simulink model "h175_model_cathode_harness_hctrl_basic"  (R2023a)
settings: Solver=VariableStepAuto  StartTime=0.0  StopTime=4750  RelTol=1e-2
InitFcn:
  | run("cathode_subsystem_parameters.m")
undefined symbols (not defined in the file or in its folder): sigbuilder_block
libraries: nesl_utility x12, fl_lib x10, simulink x5, slpidlib x2, eeGeneralControl x2, VariableTimeLowPassFilter x1
(part 1 of 2)
settings Model: Creator=adrian.taveras  LastModifiedBy=stefan.notter
settings SolverCC: MaxConsecutiveMinStep=20  ZeroCrossAlgorithm=Adaptive  DecoupledContinuousIntegration=on
settings DataIOCC: Refine=2
settings OptimizationCC: ReuseModelBlockBuffer=off
settings DebuggingCC: IgnoredZcDiagnostic=none
settings SimscapeCC: SimscapeLogType=all

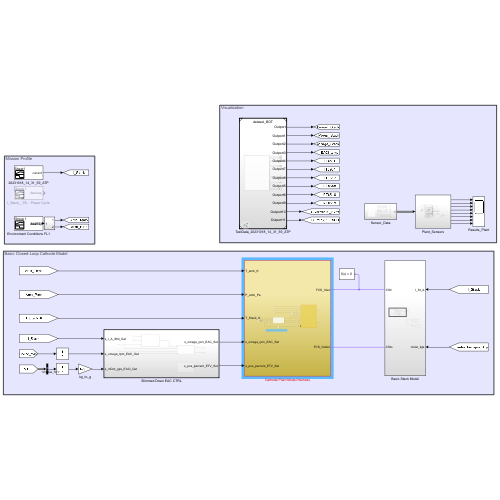
[thumbnail: Simulink's stored preview of the top-level diagram]
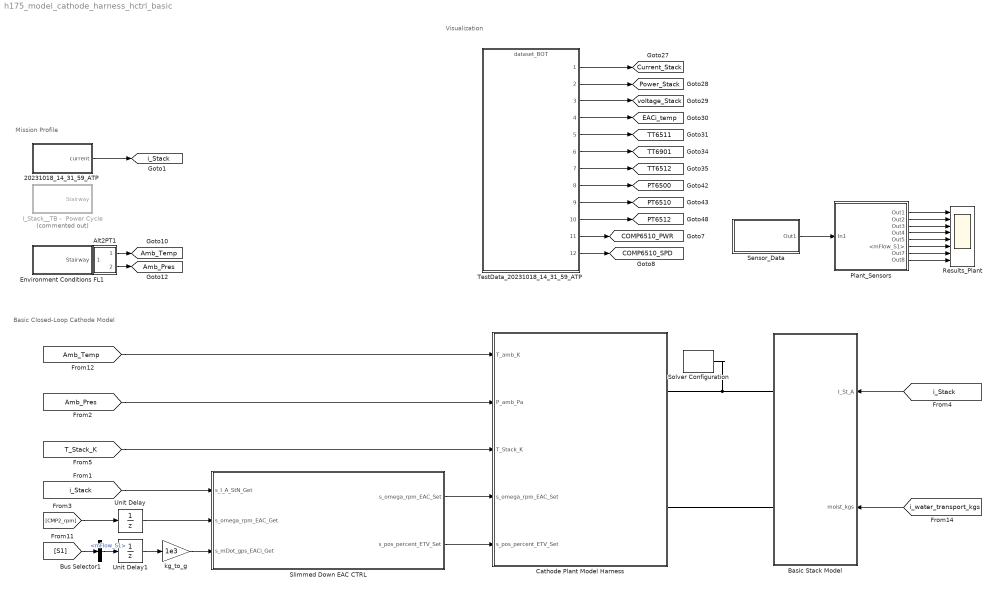
== system h175_model_cathode_harness_hctrl_basic ==
  note: Basic Closed-Loop Cathode Model
  note: Visualization
  note: Mission Profile
  20231018_14_31_59_ATP : Subsystem  Tag=STV Subsys  LoadFcn=sigbuilder_block('load');  StartFcn=sigbuilder_block('start');  StopFcn=sigbuilder_block('stop');  ClipboardFcn=sigbuilder_block('clipboard');  mask(Sigbuilder block){tuvar=[0:10]}
      mask help: Simulink:masks:SigbuilderBlock_MD
      mask init:
      | if ~strcmp(get_param(bdroot(gcbh),'SimulationStatus'),'stopped') tuvar = sigbuilder_block('maskInit'); end
      settings: CopyFcn=sigbuilder_block('copy');  DeleteFcn=sigbuilder_block('delete');  ModelCloseFcn=sigbuilder_block('modelClose');  PreSaveFcn=sigbuilder_block('preSave');  PauseFcn=sigbuilder_block('pause');  ContinueFcn=sigbuilder_block('continue');  NameChangeFcn=sigbuilder_block('namechange');  OpenFcn=sigbuilder_block('open',[725.25 330.75 938.25 556.5 ]);  CloseFcn=sigbuilder_block('close');
      mask Display: plot(0, 0, 100, 100,[2, 2, 32, 32, 2], [68, 8, 8, 68, 68],[32, 2], [38, 38], [32, 19, 2],[53, 60, 44], [32, 17, 17, 2],[16, 16, 31, 31]);txt = getActiveGroup(gcbh);text(2, 100, txt,'verticalAlignment', 'top');
  Alt2PT1 : Subsystem
  Basic Stack Model : Subsystem
      settings: PortSchema="{\"entries\":[{\"content\":{\"sides\":[{\"content\":{\"connectorIds\":[\"LConn1\",\"LConn2\"]},\"type\":\"ConnectorPlacement.EquallySpacedRectSide\",\"uuid\":\"19460938-b288-4d21-b4cd-9dae603c1776\"},{\"content\":{\"connectorIds\":[\"In1\",\"In2\"],\"side\":\"RIGHT\"},\"type\":\"ConnectorPlacement.EquallySpacedRectSide\",\"uuid\":\"f9fd6515-5c99-4012-9e0e-a9d1faf30c36\"},{\"content\":{\"side\":\"TOP\"},\"type\":\"ConnectorPlacement.EquallySpacedRectSide\",\"uuid\":\"36dd5767-135b-4114-983d-9ffe53efa4e0\"}]},\"type\":\"ConnectorPlacement.EquallySpacedConnector\",\"uuid\":\"78d4a12b-2c5e-427b-baa6-4f95f1f393d1\"}],\"packageUris\":[\"http://schema.mathworks.com/mf0/Connector/R2020b\"],\"version\":\"1.0\"}"
  Bus Selector1 : BusSelector  OutputSignals=mFlow_S1
  Cathode Plant Model Harness : Subsystem
  Environment Conditions FL1 : Subsystem  Tag=STV Subsys  LoadFcn=sigbuilder_block('load',[5.4 5.4 1141.2 580.8 ]);  StartFcn=sigbuilder_block('start');  StopFcn=sigbuilder_block('stop');  ClipboardFcn=sigbuilder_block('clipboard');  mask(Sigbuilder block){tuvar=[0:10]}
      mask help: Simulink:masks:SigbuilderBlock_MD
      mask init:
      | if ~strcmp(get_param(bdroot(gcbh),'SimulationStatus'),'stopped') tuvar = sigbuilder_block('maskInit'); end
      settings: CopyFcn=sigbuilder_block('copy');  DeleteFcn=sigbuilder_block('delete');  ModelCloseFcn=sigbuilder_block('modelClose');  PreSaveFcn=sigbuilder_block('preSave');  PauseFcn=sigbuilder_block('pause');  ContinueFcn=sigbuilder_block('continue');  NameChangeFcn=sigbuilder_block('namechange');  OpenFcn=sigbuilder_block('open',[6 30 1908 951.75 ]);  CloseFcn=sigbuilder_block('close');
      mask Display: plot(0, 0, 100, 100,[2, 2, 32, 32, 2], [68, 8, 8, 68, 68],[32, 2], [38, 38], [32, 19, 2],[53, 60, 44], [32, 17, 17, 2],[16, 16, 31, 31]);txt = getActiveGroup(gcbh);text(2, 100, txt,'verticalAlignment', 'top');
  I_Stack__TB -  Power Cycle : Subsystem  Tag=STV Subsys  Commented=on  LoadFcn=sigbuilder_block('load');  StartFcn=sigbuilder_block('start');  StopFcn=sigbuilder_block('stop');  ClipboardFcn=sigbuilder_block('clipboard');  mask(Sigbuilder block){tuvar=[0:10]}
      mask help: Simulink:masks:SigbuilderBlock_MD
      mask init:
      | if ~strcmp(get_param(bdroot(gcbh),'SimulationStatus'),'stopped') tuvar = sigbuilder_block('maskInit'); end
      settings: CopyFcn=sigbuilder_block('copy');  DeleteFcn=sigbuilder_block('delete');  ModelCloseFcn=sigbuilder_block('modelClose');  PreSaveFcn=sigbuilder_block('preSave');  PauseFcn=sigbuilder_block('pause');  ContinueFcn=sigbuilder_block('continue');  NameChangeFcn=sigbuilder_block('namechange');  OpenFcn=sigbuilder_block('open',[329.4 141 551.4 321 ]);  CloseFcn=sigbuilder_block('close');
      mask Display: plot(0, 0, 100, 100,[2, 2, 32, 32, 2], [68, 8, 8, 68, 68],[32, 2], [38, 38], [32, 19, 2],[53, 60, 44], [32, 17, 17, 2],[16, 16, 31, 31]);txt = getActiveGroup(gcbh);text(2, 100, txt,'verticalAlignment', 'top');
  Plant_Sensors : Subsystem
  Results_Plant : Scope  NumInputPorts=8
  Sensor_Data : Subsystem
  Slimmed Down EAC CTRL : Subsystem  TreatAsAtomicUnit=on
      settings: RTWFcnNameOpts=Use subsystem name  RTWFileNameOpts=Use subsystem name
  Solver Configuration : nesl_utility/Solver Configuration  PhysicalDomain=network_engine_domain  SubClassName=solver  LeftPortType=input  RightPortType=generic  Tones=[]  Harmonics=[]  SimulateNoise=off  Profile=off  UseLocalSampling=off  EnableSwitchedLinearOptims=on  FrequencyDomain=off  UseCCode=off  RelTol=0.001  AbsTol=0.001  MinStep=1e-09  ToWorkspace=off  RevertToSquareIcSolve=off  NumHomotopyIterations=100  PhasorMode=off  PhasorModeNumHarmonics=1  ConsistencySolver=NEWTON_XTOL_AFTER_FTOL  IndexReductionMethod=DerivativeReplacement  DoDC=off  ResidualTolerance=1e-09  ConsistencyTolSource=GLOBAL  ConsistencyAbsTol=0.01  ConsistencyRelTol=0.01  ConsistencyTolFactor=0.1  UseLocalSolver=off  LocalSolverChoice=NE_BACKWARD_EULER_ADVANCER  ResolveIndetEquations=on  FunctionEvalNumThread=1  LocalSolverSampleTime=0.001  DoFixedCost=off  MaxNonlinIter=3  MaxModeIter=2  ComputeImpulses=off  ImpulseIterations=2  LinearAlgebra=auto  LinearAlgebraNumThread=0  EquationFormulation=NE_TIME_EF  DelaysMemoryBudget=8096  AutomaticFiltering=on  FilteringTimeConstant=0.005  PartitionStorageMethod=AS_NEEDED  PartitionMemoryBudget=1024  PartitionMethod=ROBUST
  TestData_20231018_14_31_59_ATP : ModelReference  ModelNameDialog=dataset_BOT.slx  SimulationMode=Normal  ModelReferenceVersion=1.7
  Unit Delay : UnitDelay  SampleTime=-1  HasFrameUpgradeWarning=on
  Unit Delay1 : UnitDelay  SampleTime=-1  HasFrameUpgradeWarning=on
  kg_to_g : Gain  Gain=1e3
  tag scope: Amb_Pres=global, Amb_Temp=global, COMP6510_PWR=global, COMP6510_SPD=global, Current_Stack=global, EACi_temp=global, PT6500=global, PT6510=global, PT6512=global, Power_Stack=global, TT6511=global, TT6512=global, TT6901=global, i_Stack=global, voltage_Stack=global
  wires:
  Plant_Sensors/1(Out1) -> Results_Plant/1
  Plant_Sensors/2(Out2) -> Results_Plant/2
  Plant_Sensors/3(Out3) -> Results_Plant/3
  Plant_Sensors/4(Out4) -> Results_Plant/4
  Plant_Sensors/5(Out5) -> Results_Plant/5
  Plant_Sensors/6(<mFlow_S1>) -> Results_Plant/6
  Plant_Sensors/7(Out7) -> Results_Plant/7
  Plant_Sensors/8(Out8) -> Results_Plant/8
  Alt2PT1/2(Out2) -> [Amb_Pres]
  Environment Conditions FL1/1(Stairway) -> Alt2PT1/1(In1)
  Alt2PT1/1(Out1) -> [Amb_Temp]
  20231018_14_31_59_ATP/1(current) -> [i_Stack]
  Sensor_Data/1(Out1) -> Plant_Sensors/1(In1)
  TestData_20231018_14_31_59_ATP/1 -> [Current_Stack]
  TestData_20231018_14_31_59_ATP/2 -> [Power_Stack]
  TestData_20231018_14_31_59_ATP/3 -> [voltage_Stack]
  TestData_20231018_14_31_59_ATP/4 -> [EACi_temp]
  TestData_20231018_14_31_59_ATP/5 -> [TT6511]
  TestData_20231018_14_31_59_ATP/6 -> [TT6901]
  TestData_20231018_14_31_59_ATP/7 -> [TT6512]
  TestData_20231018_14_31_59_ATP/11 -> [COMP6510_PWR]
  TestData_20231018_14_31_59_ATP/12 -> [COMP6510_SPD]
  TestData_20231018_14_31_59_ATP/10 -> [PT6512]
  TestData_20231018_14_31_59_ATP/9 -> [PT6510]
  TestData_20231018_14_31_59_ATP/8 -> [PT6500]
  [i_Stack] -> Basic Stack Model/1(I_St_A)
  [i_water_transport_kgs] -> Basic Stack Model/2(moist_kgs)
  [Amb_Temp] -> Cathode Plant Model Harness/1(T_amb_K)
  [Amb_Pres] -> Cathode Plant Model Harness/2(P_amb_Pa)
  Slimmed Down EAC CTRL/1(s_omega_rpm_EAC_Set) -> Cathode Plant Model Harness/4(s_omega_rpm_EAC_Set)
  Slimmed Down EAC CTRL/2(s_pos_percent_ETV_Set) -> Cathode Plant Model Harness/5(s_pos_percent_ETV_Set)
  [i_Stack] -> Slimmed Down EAC CTRL/1(s_I_A_StN_Get)
  [CMP2_rpm] -> Unit Delay/1
  [S1] -> Bus Selector1/1
  Bus Selector1/1 -> Unit Delay1/1  "<mFlow_S1>"
  kg_to_g/1 -> Slimmed Down EAC CTRL/3(s_mDot_gps_EACi_Get)
  Unit Delay/1 -> Slimmed Down EAC CTRL/2(s_omega_rpm_EAC_Get)
  Unit Delay1/1 -> kg_to_g/1
  [T_Stack_K] -> Cathode Plant Model Harness/3(T_Stack_K)
  connections:
  Solver Configuration/RConn1 -- Basic Stack Model/LConn1 -- Cathode Plant Model Harness/RConn1
  Basic Stack Model/LConn2 -- Cathode Plant Model Harness/RConn2

== system h175_model_cathode_harness_hctrl_basic/20231018_14_31_59_ATP ==
  Demux : Demux  Tag=STV Demux  Outputs=1
      settings: DisplayOption=none
  FromWs : FromWorkspace  Tag=STV FromWs  VariableName=tuvar
      SigBuilderData=|
      | common.afterFinalStr = 'Extrapolate'
      | common.sampleTime = 0
      | dataSet.timeRange = [0 4735]
      | dataSet.name = 'Sheet1'
      | sbobj.Groups.Name = 'Sheet1'
      | sbobj.Groups.Signals.Name = 'current'
      | sbobj.Groups.Signals.XData = [0 710 730 830 850 1000 1020 1080 1100 1200 1230 1260 1270 1320 1340 1390 1405 1455 1475 1525 1565 3990 4000 4030 4090 4130 4245 4270 4345 4355 4385 4395 4735]
      | sbobj.Groups.Signals.YData = [5 5 45 45 100 100 200 200 300 300 45 45 50 50 200 200 300 300 100 100 420 420 340 420 260 340 340 50 50 45 45 5 5]
      | sbobj.Groups.TimeRange = [0 4735]
  current : Outport  Tag=STV Outport
  wires:
  Demux/1 -> current/1
  FromWs/1 -> Demux/1

== system h175_model_cathode_harness_hctrl_basic/Alt2PT1 ==
  In1 : Inport
  Add1 : Sum  Inputs=-+
  Constant4 : Constant  Value=0.0065
  Constant5 : Constant  Value=288.15
  Constant6 : Constant  Value=101330
  Constant7 : Constant  Value=4.256
  Constant8 : Constant  Value=288.15
  Divide1 : Product  Inputs=*/
  Math Function1 : Math  Operator=pow
  Product2 : Product
  Product3 : Product
  Out1 : Outport
  Out2 : Outport  Port=2
  wires:
  Constant5/1 -> Divide1/2
  Constant8/1 -> Add1/2
  In1/1 -> Product2/1
  Add1/1 -> Out1/1, Divide1/1
  Constant4/1 -> Product2/2
  Math Function1/1 -> Product3/1
  Constant7/1 -> Math Function1/2
  Divide1/1 -> Math Function1/1
  Product2/1 -> Add1/1
  Constant6/1 -> Product3/2
  Product3/1 -> Out2/1

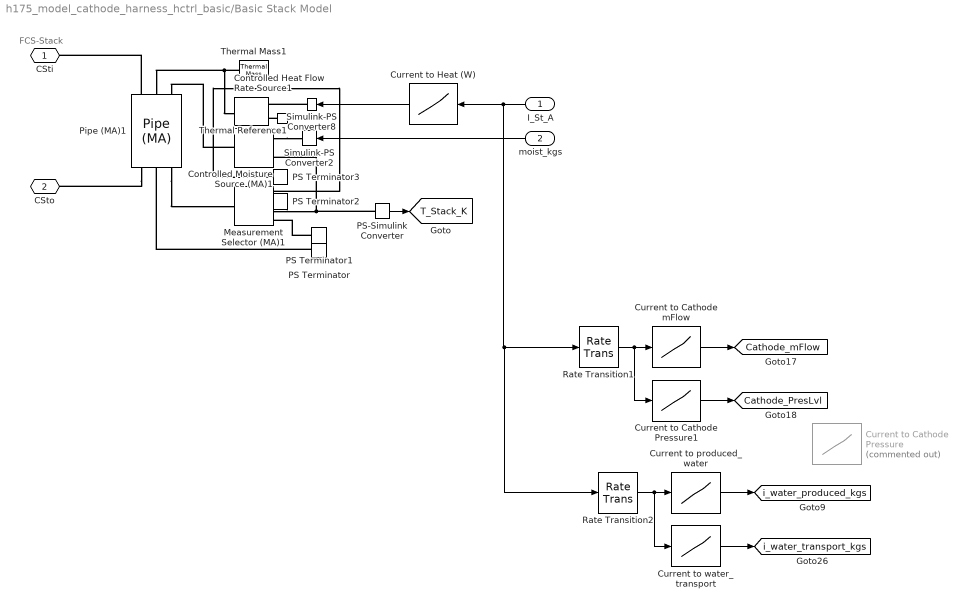
== system h175_model_cathode_harness_hctrl_basic/Basic Stack Model ==
  note: FCS-Stack
  I_St_A : Inport
  moist_kgs : Inport  Port=2
  Controlled Heat Flow Rate Source1 : fl_lib/Thermal/Thermal Sources/Controlled Heat Flow Rate Source
  Controlled Moisture Source (MA)1 : fl_lib/Moist Air/Sources/Moisture & Trace Gas Sources/Controlled Moisture Source (MA)  moisture_source_spec=foundation.enum.moisture_source_spec.vapor  Phi_S_specify=off  Phi_S_priority=None  Phi_S=0 kW  Phi_S_nominal_specify=off  Phi_S_nominal_unit=kW  Phi_S_nominal_value=1  mdot_w_S_specify=off  mdot_w_S_priority=None  mdot_w_S=0 kg/s  mdot_w_S_nominal_specify=off  mdot_w_S_nominal_unit=kg/s  mdot_w_S_nominal_value=1
      settings: InternalSimscapePortConfiguration="{\"Bottom\":[],\"Left\":[{\"id\":\"S\",\"label\":\"S\",\"type\":\"foundation.moist_air.moist_air_source\"}],\"Right\":[{\"id\":\"M\",\"label\":\"M\",\"type\":\"input\"},{\"id\":\"T\",\"label\":\"T\",\"type\":\"input\"}],\"Top\":[]}"
  Current to Cathode Pressure : Lookup_n-D  Commented=on  NumberOfTableDimensions=1  BreakpointsForDimension1=[0;50;100;150;200;250;300;350;400;510;600]  Table=[101330;110000;115000;125000;130000;140000;150000;165000;180000;200000;230000]  InternalRulePriority=Speed  RndMeth=Simplest
  Current to Cathode Pressure1 : Lookup_n-D  NumberOfTableDimensions=1  BreakpointsForDimension1=[0;50;100;150;200;250;300;350;400;510;600]  Table=[101330;140000;150000;175000;185000;195000;202500;210000;220000;235000;250000]  InternalRulePriority=Speed  RndMeth=Simplest
  Current to Cathode mFlow : Lookup_n-D  NumberOfTableDimensions=1  BreakpointsForDimension1=[0;50;100;150;200;250;300;350;400;510;600]  Table=[0;0.01;0.0225;0.035;0.045;0.055;0.068;0.0825;0.1;0.135;0.167]  InternalRulePriority=Speed  RndMeth=Simplest
  Current to Heat (W) : Lookup_n-D  NumberOfTableDimensions=1  BreakpointsForDimension1=[0:50:400]  Table=[0, 9932, 21438, 33442,47123, 59491, 77033, 93585, 112042]  InternalRulePriority=Speed  RndMeth=Simplest
  Current to produced_water : Lookup_n-D  NumberOfTableDimensions=1  BreakpointsForDimension1=[0;100;200;400;600]  Table=[0;6.491e-6;1.132e-5;1.762e-5;2.762e-5]  InternalRulePriority=Speed  RndMeth=Simplest
  Current to water_transport : Lookup_n-D  NumberOfTableDimensions=1  BreakpointsForDimension1=[0;100;200;400;600]  Table=[0;4.247e-3;8.494e-3;1.697e-2;2.548e-2]  InternalRulePriority=Speed  RndMeth=Simplest
  Measurement Selector (MA)1 : fl_lib/Moist Air/Sensors/Measurement Selector (MA)  moisture_spec=foundation.enum.moisture_spec.relative_humidity  trace_gas_spec=foundation.enum.trace_gas_spec.mole_fraction
  PS Terminator{,1..3} (4 alike) : fl_lib/Physical Signals/Sinks/PS Terminator
  PS-Simulink Converter : nesl_utility/PS-Simulink Converter  PhysicalDomain=network_engine_domain  SubClassName=ps_output  LeftPortType=input  RightPortType=output  PseudoPeriodic=off  Frequencies=[]  VectorFormat=inherit  Unit=inherit  AffineConversion=off
  Pipe (MA)1 : fl_lib/Moist Air/Elements/Pipe (MA)  length=1 m  area=1 m^2  Dh=.1 m  length_add=.1 m  roughness=15e-6 m  Re_lam=2000  Re_tur=4000  shape_factor=1  Nu_lam=3.66  wall_condensation=simscape.enum.onoff.on  RH_ws=1  time_constant=1e-3 s  moisture_trace_gas_source=foundation.enum.moisture_trace_gas_source.controlled  moisture_source_spec=foundation.enum.moisture_source_spec.vapor  moisture_mass_flow=0 kg/s  moisture_temperature_spec=foundation.enum.temperature_spec.atmospheric  moisture_temperature=293.15 K  trace_gas_mass_flow=0 kg/s  trace_gas_temperature_spec=foundation.enum.temperature_spec.atmospheric  trace_gas_temperature=293.15 K  p_I_specify=off  p_I_priority=High  p_I=0.101325 MPa  p_I_nominal_specify=off  p_I_nominal_unit=MPa  p_I_nominal_value=1  T_I_specify=off  T_I_priority=High  T_I=293.15 K  T_I_nominal_specify=off  T_I_nominal_unit=K  T_I_nominal_value=1  RH_I_specify=off  RH_I_priority=High  RH_I=0  RH_I_nominal_specify=off  RH_I_nominal_unit=1  RH_I_nominal_value=1  x_w_I_specify=off  x_w_I_priority=None  x_w_I=0  x_w_I_nominal_specify=off  x_w_I_nominal_unit=1  x_w_I_nominal_value=1  y_w_I_specify=off  y_w_I_priority=None  y_w_I=0  y_w_I_nominal_specify=off  y_w_I_nominal_unit=1  y_w_I_nominal_value=1  HR_I_specify=off  HR_I_priority=None  HR_I=0  HR_I_nominal_specify=off  HR_I_nominal_unit=1  HR_I_nominal_value=1  x_g_I_specify=off  x_g_I_priority=High  x_g_I=0  x_g_I_nominal_specify=off  x_g_I_nominal_unit=1  x_g_I_nominal_value=1  y_g_I_specify=off  y_g_I_priority=None  y_g_I=0  y_g_I_nominal_specify=off  y_g_I_nominal_unit=1  y_g_I_nominal_value=1
      settings: InternalSimscapePortConfiguration="{\"Bottom\":[],\"Left\":[{\"id\":\"A\",\"label\":\"A\",\"type\":\"foundation.moist_air.moist_air\"},{\"id\":\"H\",\"label\":\"H\",\"type\":\"foundation.thermal.thermal\"},{\"id\":\"S\",\"label\":\"S\",\"type\":\"foundation.moist_air.moist_air_source\"}],\"Right\":[{\"id\":\"B\",\"label\":\"B\",\"type\":\"foundation.moist_air.moist_air\"},{\"id\":\"W\",\"label\":\"W\",\"type\":\"output\"},{\"id\":\"F\",\"label\":\"F\",\"type\":\"output\"}],\"Top\":[]}"
  Rate Transition1 : RateTransition
  Rate Transition2 : RateTransition
  Simulink-PS Converter2 : nesl_utility/Simulink-PS Converter  PhysicalDomain=network_engine_domain  SubClassName=ps_input  LeftPortType=input  RightPortType=output  PseudoPeriodic=off  Frequencies=[]  NoiseDistribution=none  NoiseParameters=[]  Unit=1  AffineConversion=off  FilteringAndDerivatives=provide  SimscapeFilterOrder=1  InputFilterTimeConstant=0.001  UdotUserProvided=0
  Simulink-PS Converter8 : nesl_utility/Simulink-PS Converter  PhysicalDomain=network_engine_domain  SubClassName=ps_input  LeftPortType=input  RightPortType=output  PseudoPeriodic=off  Frequencies=[]  NoiseDistribution=none  NoiseParameters=[]  Unit=W  AffineConversion=off  FilteringAndDerivatives=provide  SimscapeFilterOrder=1  InputFilterTimeConstant=0.001  UdotUserProvided=0
  Thermal Mass1 : fl_lib/Thermal/Thermal Elements/Thermal Mass  mass_type=foundation.enum.constant_variable.constant  mass=10 kg  sp_heat=447 J/(K*kg)  mass_min=1e-6 kg  num_ports=foundation.enum.numPorts2.one  m_specify=off  m_priority=High  m=1 kg  m_nominal_specify=off  m_nominal_unit=kg  m_nominal_value=1  T_specify=off  T_priority=High  T=300 K  T_nominal_specify=off  T_nominal_unit=K  T_nominal_value=1  Q_specify=off  Q_priority=None  Q=0 W  Q_nominal_specify=off  Q_nominal_unit=W  Q_nominal_value=1
  Thermal Reference1 : fl_lib/Thermal/Thermal Elements/Thermal Reference
  CSti : PMIOPort  Side=Left
  CSto : PMIOPort  Port=2  Side=Left
  tag scope: Cathode_PresLvl=global, Cathode_mFlow=global, T_Stack_K=global, i_water_produced_kgs=global, i_water_transport_kgs=global
  wires:
  Current to Heat (W)/1 -> Simulink-PS Converter8/1
  moist_kgs/1 -> Simulink-PS Converter2/1
  I_St_A/1 -> Current to Heat (W)/1, Rate Transition2/1, Rate Transition1/1
  Rate Transition2/1 -> Current to water_transport/1, Current to produced_water/1
  Current to Cathode Pressure1/1 -> [Cathode_PresLvl]
  Current to water_transport/1 -> [i_water_transport_kgs]
  Rate Transition1/1 -> Current to Cathode Pressure1/1, Current to Cathode mFlow/1
  Current to Cathode mFlow/1 -> [Cathode_mFlow]
  Current to produced_water/1 -> [i_water_produced_kgs]
  PS-Simulink Converter/1 -> [T_Stack_K]
  connections:
  Measurement Selector (MA)1/RConn2 -- PS-Simulink Converter/LConn1 -- Controlled Moisture Source (MA)1/RConn2
  Thermal Mass1/LConn1 -- Controlled Heat Flow Rate Source1/LConn1 -- Pipe (MA)1/LConn2
  PS Terminator3/LConn1 -- Measurement Selector (MA)1/RConn4
  Thermal Reference1/LConn1 -- Controlled Heat Flow Rate Source1/RConn2
  Controlled Moisture Source (MA)1/RConn1 -- Simulink-PS Converter2/RConn1
  Pipe (MA)1/RConn3 -- Measurement Selector (MA)1/LConn1
  Controlled Moisture Source (MA)1/LConn1 -- Pipe (MA)1/LConn3
  Simulink-PS Converter8/RConn1 -- Controlled Heat Flow Rate Source1/RConn1
  Pipe (MA)1/LConn1 -- CSti/RConn1
  PS Terminator1/LConn1 -- Measurement Selector (MA)1/RConn1
  PS Terminator2/LConn1 -- Measurement Selector (MA)1/RConn3
  Pipe (MA)1/RConn1 -- CSto/RConn1
  PS Terminator/LConn1 -- Pipe (MA)1/RConn2

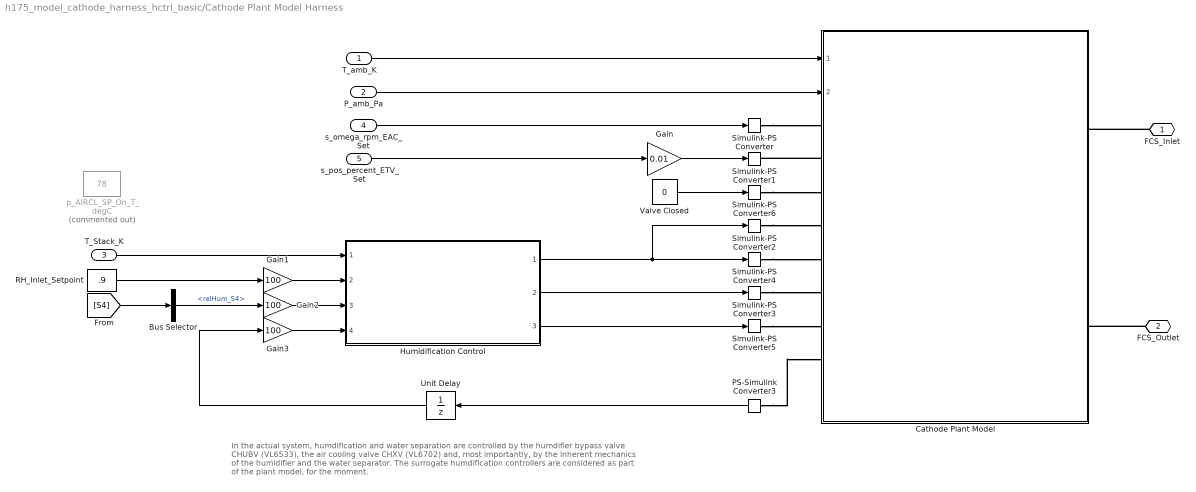
== system h175_model_cathode_harness_hctrl_basic/Cathode Plant Model Harness ==
  note: In the actual system, humdification and water separation are controlled by the humdifier bypass valve CHUBV (VL6533), the air cooling valve CHXV (VL6702) and, most importantly, by the inherent mechanics of the humidifier and the water separator.
      | The surrogate humdification controllers are considered as part of the plant model, for the moment.
  T_amb_K : Inport
  P_amb_Pa : Inport  Port=2
  T_Stack_K : Inport  Port=3
  s_omega_rpm_EAC_Set : Inport  Port=4
  s_pos_percent_ETV_Set : Inport  Port=5
  Bus Selector : BusSelector  OutputSignals=relHum_S4
  Cathode Plant Model : Subsystem  ReferencedSubsystem=cathode_subsystem_model
      settings: PortSchema="{\"entries\":[{\"content\":{\"sides\":[{\"content\":{\"connectorIds\":[\"In1\",\"In2\",\"LConn8\",\"LConn9\",\"LConn7\",\"LConn1\",\"LConn4\",\"LConn2\",\"LConn3\",\"LConn5\",\"LConn6\"]},\"type\":\"ConnectorPlacement.EquallySpacedRectSide\",\"uuid\":\"e3b30cb5-20d3-4977-927f-9fea068a9234\"},{\"content\":{\"connectorIds\":[\"RConn1\",\"RConn2\"],\"side\":\"RIGHT\"},\"type\":\"ConnectorPlacement.EquallySpacedRectSide\",\"uuid\":\"2d547627-9665-492a-afa4-fcc16b1173a1\"},{\"content\":{\"side\":\"TOP\"},\"type\":\"ConnectorPlacement.EquallySpacedRectSide\",\"uuid\":\"4ee6a80a-af1f-40b1-aa59-916ec7fe1294\"}]},\"type\":\"ConnectorPlacement.EquallySpacedConnector\",\"uuid\":\"0d82e4d1-cc18-4647-90fc-0df577891cdc\"}],\"packageUris\":[\"http://schema.mathworks.com/mf0/Connector/R2020b\"],\"version\":\"1.0\"}"
  Gain : Gain  Gain=0.01
  Gain1 : Gain  Gain=100
  Gain2 : Gain  Gain=100
  Gain3 : Gain  Gain=100
  Humidification Control : Subsystem  ReferencedSubsystem=cathode_subsystem_humdification
  PS-Simulink Converter3 : nesl_utility/PS-Simulink Converter  PhysicalDomain=network_engine_domain  SubClassName=ps_output  LeftPortType=input  RightPortType=output  PseudoPeriodic=off  Frequencies=[]  VectorFormat=inherit  Unit=inherit  AffineConversion=off
  RH_Inlet_Setpoint : Constant  Value=.9
  Simulink-PS Converter{,1..6} (7 alike) : nesl_utility/Simulink-PS Converter  PhysicalDomain=network_engine_domain  SubClassName=ps_input  LeftPortType=input  RightPortType=output  PseudoPeriodic=off  Frequencies=[]  NoiseDistribution=none  NoiseParameters=[]  Unit=1  AffineConversion=off  FilteringAndDerivatives=provide  SimscapeFilterOrder=1  InputFilterTimeConstant=0.001  UdotUserProvided=0
  Unit Delay : UnitDelay  SampleTime=-1  HasFrameUpgradeWarning=on
  Valve Closed : Constant  Value=0
  p_AIRCL_SP_On_T_degC : Constant  Commented=on  Value=78
  FCS_Inlet : PMIOPort  Side=Right
  FCS_Outlet : PMIOPort  Port=2  Side=Right
  wires:
  T_amb_K/1 -> Cathode Plant Model/1
  P_amb_Pa/1 -> Cathode Plant Model/2
  s_omega_rpm_EAC_Set/1 -> Simulink-PS Converter/1
  s_pos_percent_ETV_Set/1 -> Gain/1
  RH_Inlet_Setpoint/1 -> Gain1/1
  T_Stack_K/1 -> Humidification Control/1
  Gain/1 -> Simulink-PS Converter1/1
  Humidification Control/3 -> Simulink-PS Converter5/1
  Humidification Control/1 -> Simulink-PS Converter4/1, Simulink-PS Converter2/1
  Humidification Control/2 -> Simulink-PS Converter3/1
  Valve Closed/1 -> Simulink-PS Converter6/1
  Gain1/1 -> Humidification Control/2
  [S4] -> Bus Selector/1
  Bus Selector/1 -> Gain2/1  "<relHum_S4>"
  Gain2/1 -> Humidification Control/3
  PS-Simulink Converter3/1 -> Unit Delay/1
  Unit Delay/1 -> Gain3/1
  Gain3/1 -> Humidification Control/4
  connections:
  FCS_Inlet/RConn1 -- Cathode Plant Model/RConn1
  FCS_Outlet/RConn1 -- Cathode Plant Model/RConn2
  Simulink-PS Converter/RConn1 -- Cathode Plant Model/LConn8
  Cathode Plant Model/LConn9 -- Simulink-PS Converter1/RConn1
  Simulink-PS Converter6/RConn1 -- Cathode Plant Model/LConn7
  Simulink-PS Converter2/RConn1 -- Cathode Plant Model/LConn1
  Simulink-PS Converter3/RConn1 -- Cathode Plant Model/LConn2
  Simulink-PS Converter4/RConn1 -- Cathode Plant Model/LConn4
  Simulink-PS Converter5/RConn1 -- Cathode Plant Model/LConn3
  PS-Simulink Converter3/LConn1 -- Cathode Plant Model/LConn5

== system h175_model_cathode_harness_hctrl_basic/Environment Conditions FL1 ==
  Demux : Demux  Tag=STV Demux  Outputs=1
      settings: DisplayOption=none
  FromWs : FromWorkspace  Tag=STV FromWs  VariableName=tuvar
      SigBuilderData=|
      | common.afterFinalStr = 'Extrapolate'
      | common.sampleTime = 0
      | dataSet.timeRange = [0 22226]
      | dataSet.name = 'Group 1'
      | sbobj.Groups.Name = 'Group 1'
      | sbobj.Groups.Signals.Name = 'Stairway'
      | sbobj.Groups.Signals.XData = [0 1 1.1 1.2 1.3 120 270 670 1450 7450 7510 21146 21826 22226]
      | sbobj.Groups.Signals.YData = [0 0 0 0 0 0 250 650 1100 1100 1000 1000 500 0]
      | sbobj.Groups.TimeRange = [0 22226]
  Stairway : Outport  Tag=STV Outport
  wires:
  Demux/1 -> Stairway/1
  FromWs/1 -> Demux/1

== system h175_model_cathode_harness_hctrl_basic/I_Stack__TB -  Power Cycle ==
  Demux : Demux  Tag=STV Demux  Outputs=1
      settings: DisplayOption=none
  FromWs : FromWorkspace  Tag=STV FromWs  VariableName=tuvar
      SigBuilderData=|
      | common.afterFinalStr = 'Extrapolate'
      | common.sampleTime = 0
      | dataSet.timeRange = [0 600]
      | dataSet.name = 'Group 1'
      | sbobj.Groups.Name = 'Group 1'
      | sbobj.Groups.Signals.Name = 'Stairway'
      | sbobj.Groups.Signals.XData = [0 180 190 250 260 320 330 390 410 460 470 530 540 600]
      | sbobj.Groups.Signals.YData = [100 100 200 200 400 400 600 600 300 300 200 200 100 100]
      | sbobj.Groups.TimeRange = [0 600]
  Stairway : Outport  Tag=STV Outport
  wires:
  Demux/1 -> Stairway/1
  FromWs/1 -> Demux/1

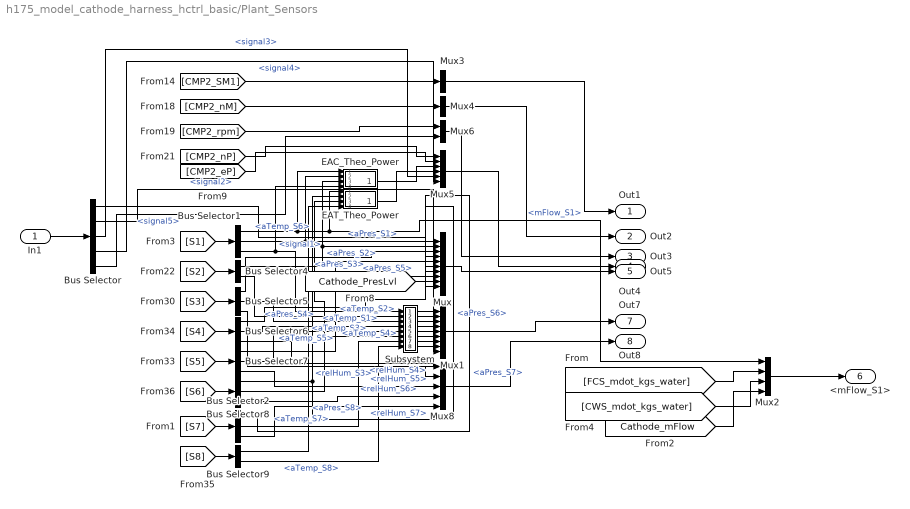
== system h175_model_cathode_harness_hctrl_basic/Plant_Sensors ==
  In1 : Inport
  Bus Selector : BusSelector  OutputSignals=signal1,signal2,signal3,signal4,signal5
  Bus Selector1 : BusSelector  OutputSignals=mFlow_S1,aPres_S1,aTemp_S1
  Bus Selector2 : BusSelector  OutputSignals=aPres_S7,aTemp_S7,relHum_S7
  Bus Selector4 : BusSelector  OutputSignals=aPres_S2,aTemp_S2
  Bus Selector5 : BusSelector  OutputSignals=aPres_S3,aTemp_S3,relHum_S3
  Bus Selector6 : BusSelector  OutputSignals=aPres_S4,aTemp_S4,relHum_S4
  Bus Selector7 : BusSelector  OutputSignals=aPres_S5,aTemp_S5,relHum_S5
  Bus Selector8 : BusSelector  OutputSignals=aPres_S6,aTemp_S6,relHum_S6
  Bus Selector9 : BusSelector  OutputSignals=aPres_S8,aTemp_S8
  EAC_Theo_Power : Subsystem
  EAT_Theo_Power : Subsystem
  Mux : Mux  Inputs=10
  Mux1 : Mux  Inputs=9
  Mux2 : Mux
  Mux3 : Mux  Inputs=1
  Mux4 : Mux  Inputs=1
  Mux5 : Mux  Inputs=6
  Mux6 : Mux  Inputs=2
  Mux8 : Mux  Inputs=5
  Subsystem : Subsystem
  Out1 : Outport
  Out2 : Outport  Port=2
  Out3 : Outport  Port=3
  Out4 : Outport  Port=4
  Out5 : Outport  Port=5
  <mFlow_S1> : Outport  Port=6
  Out7 : Outport  Port=7
  Out8 : Outport  Port=8
  wires:
  [CMP2_eP] -> Mux5/2
  [CMP2_nP] -> Mux5/1
  Mux3/1 -> Out1/1
  [S8] -> Bus Selector9/1
  [CMP2_SM1] -> Mux3/1
  Bus Selector7/3 -> Mux8/3  "<relHum_S5>"
  Bus Selector9/1 -> EAT_Theo_Power/4(<aPres_S7>), Mux/8  "<aPres_S8>"
  Bus Selector4/1 -> EAC_Theo_Power/3(<aPres_S2>), Mux/2  "<aPres_S2>"
  [CMP2_rpm] -> Mux6/1
  [CMP2_nM] -> Mux4/1
  Bus Selector6/1 -> Mux/4  "<aPres_S4>"
  [S5] -> Bus Selector7/1
  Mux/1 -> Out5/1
  Bus Selector5/3 -> Mux8/1  "<relHum_S3>"
  Bus Selector5/1 -> Mux/3  "<aPres_S3>"
  [S4] -> Bus Selector6/1
  Mux6/1 -> Out3/1
  [S3] -> Bus Selector5/1
  Bus Selector1/1 -> Mux2/1, EAT_Theo_Power/1(<mFlow_S1>), EAC_Theo_Power/1(<mFlow_S1>)  "<mFlow_S1>"
  Bus Selector7/1 -> Mux/5  "<aPres_S5>"
  Bus Selector8/1 -> EAT_Theo_Power/2(<aPres_S6>), Mux/6  "<aPres_S6>"
  [S1] -> Bus Selector1/1
  [Cathode_PresLvl] -> Mux/9
  Mux5/1 -> Out4/1
  Bus Selector6/3 -> Mux8/2  "<relHum_S4>"
  Bus Selector8/3 -> Mux8/4  "<relHum_S6>"
  [S6] -> Bus Selector8/1
  Bus Selector1/2 -> Mux/1, EAC_Theo_Power/2(<aPres_S1>)  "<aPres_S1>"
  [S2] -> Bus Selector4/1
  Mux4/1 -> Out2/1
  Mux1/1 -> Out7/1
  Mux8/1 -> Out8/1
  Bus Selector1/3 -> EAC_Theo_Power/4(<aTemp_S1>), Subsystem/1(<aTemp_S1>)  "<aTemp_S1>"
  Bus Selector4/2 -> Subsystem/2(<aTemp_S2>)  "<aTemp_S2>"
  Bus Selector5/2 -> Subsystem/3(<aTemp_S3>)  "<aTemp_S3>"
  Bus Selector6/2 -> Subsystem/4(<aTemp_S4>)  "<aTemp_S4>"
  Bus Selector7/2 -> Subsystem/5(<aTemp_S5>)  "<aTemp_S5>"
  Bus Selector8/2 -> EAT_Theo_Power/3(<aTemp_S6>), Subsystem/6(<aTemp_S6>)  "<aTemp_S6>"
  Bus Selector9/2 -> Subsystem/8(<aTemp_S7>)  "<aTemp_S8>"
  Subsystem/1(Out1) -> Mux1/1
  Subsystem/2(Out2) -> Mux1/2
  Subsystem/3(Out3) -> Mux1/3
  Subsystem/4(Out4) -> Mux1/4
  Subsystem/5(Out5) -> Mux1/5
  Subsystem/6(Out6) -> Mux1/6
  Subsystem/7(Out7) -> Mux1/7
  EAC_Theo_Power/1(Out1) -> Mux5/3
  EAT_Theo_Power/1(Out1) -> Mux5/4
  [S7] -> Bus Selector2/1
  Bus Selector2/2 -> Subsystem/7(In8)  "<aTemp_S7>"
  Subsystem/8(Out8) -> Mux1/8
  Bus Selector2/1 -> Mux/7  "<aPres_S7>"
  Bus Selector2/3 -> Mux8/5  "<relHum_S7>"
  [FCS_mdot_kgs_water] -> Mux2/2
  Mux2/1 -> <mFlow_S1>/1
  [Cathode_mFlow] -> Mux2/4
  [CWS_mdot_kgs_water] -> Mux2/3
  In1/1 -> Bus Selector/1
  Bus Selector/1 -> Mux/10  "<signal1>"
  Bus Selector/2 -> Mux1/9  "<signal2>"
  Bus Selector/5 -> Mux6/2  "<signal5>"
  Bus Selector/3 -> Mux5/5  "<signal3>"
  Bus Selector/4 -> Mux5/6  "<signal4>"

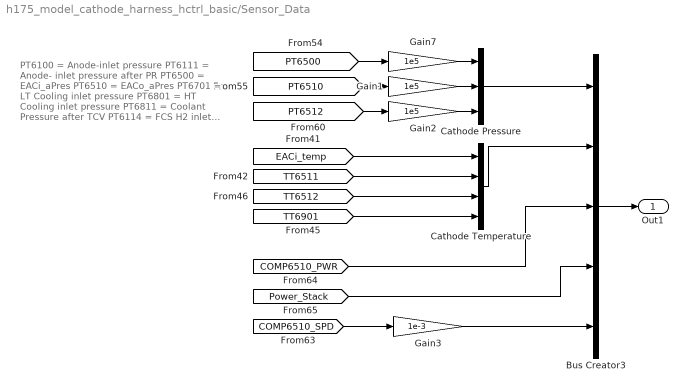
== system h175_model_cathode_harness_hctrl_basic/Sensor_Data ==
  note: PT6100 = Anode-inlet pressure
      | PT6111 = Anode- inlet pressure after PR
      | PT6500 = EACi_aPres
      | PT6510 = EACo_aPres
      | PT6701 = LT Cooling inlet pressure
      | PT6801 = HT Cooling inlet pressure
      | PT6811 = Coolant Pressure after TCV
      | PT6114 = FCS H2 inlet pressure
      | PT6512 = FCS O2 inlet Pressure
      | PT6812 = FCS Coolant inlet pressure
      |
      | TT6100 = Anode- inlet Temperature
      | TT6111 = Anode- after Temperature
      | TT6500 = EACi_Temp
      | TT6510 = EACo_Temp
      | TT6701 = LT Cooling inlet Temperature
      | TT6801 = HT Cooling inlet Temperature
      | TT6811 = Coolant Temperature after TCV
      | TT6114 = FCS H2 inlet Temperature
      | TT6512 = FCS O2 inlet Temperature
      | TT6812 = FCS Coolant inlet Temperature
  Bus Creator3 : BusCreator  Inputs=5
  Cathode Pressure : Mux  Inputs=3
  Cathode Temperature : Mux
  Gain1 : Gain  Gain=1e5
  Gain2 : Gain  Gain=1e5
  Gain3 : Gain  Gain=1e-3
  Gain7 : Gain  Gain=1e5
  Out1 : Outport
  wires:
  Gain7/1 -> Cathode Pressure/1
  [PT6500] -> Gain7/1
  [PT6510] -> Gain1/1
  [COMP6510_SPD] -> Gain3/1
  [Power_Stack] -> Bus Creator3/4
  [COMP6510_PWR] -> Bus Creator3/3
  [PT6512] -> Gain2/1
  Gain1/1 -> Cathode Pressure/2
  [EACi_temp] -> Cathode Temperature/1
  [TT6511] -> Cathode Temperature/2
  Gain2/1 -> Cathode Pressure/3
  [TT6901] -> Cathode Temperature/4
  [TT6512] -> Cathode Temperature/3
  Cathode Pressure/1 -> Bus Creator3/1
  Cathode Temperature/1 -> Bus Creator3/2
  Bus Creator3/1 -> Out1/1
  Gain3/1 -> Bus Creator3/5

== system h175_model_cathode_harness_hctrl_basic/Slimmed Down EAC CTRL ==
  s_I_A_StN_Get : Inport
  s_omega_rpm_EAC_Get : Inport  Port=2
  s_mDot_gps_EACi_Get : Inport  Port=3
  "1: Const. Massflow, 2: Current-Based" : Constant  Value=2
  FischerWithTurbineControl : Subsystem  TreatAsAtomicUnit=on  VariantControl=variantConfig.EAC == VARIANT_EAC.FischerWithTurbine
  Subsystem : Subsystem
  TurbineDrainSequencing : Subsystem  Commented=on
  p_EAC_SP_ConstMassflow_mDot_gps : Constant  Value=30
  s_omega_rpm_EAC_Set : Outport
  s_pos_percent_ETV_Set : Outport  Port=2
  wires:
  Subsystem/1(s_EAC_mDotSP_gps) -> FischerWithTurbineControl/1(s_EAC_mDotSP_gps)
  p_EAC_SP_ConstMassflow_mDot_gps/1 -> Subsystem/2(s_EAC_SP_ConstMassflow_mDot_ps)
  "1: Const. Massflow, 2: Current-Based"/1 -> Subsystem/1(s_EAC_CurrentState_enum)
  s_I_A_StN_Get/1 -> Subsystem/3(s_I_A_StN_Get), FischerWithTurbineControl/2(s_I_A_StN_Get)
  s_omega_rpm_EAC_Get/1 -> FischerWithTurbineControl/3(s_omega_rpm_EAC_Get)
  s_mDot_gps_EACi_Get/1 -> FischerWithTurbineControl/4(s_mDot_gps_EACi_Get)
  FischerWithTurbineControl/1(s_omega_rpm_EAC_Set) -> s_omega_rpm_EAC_Set/1
  FischerWithTurbineControl/2(s_pos_percent_ETV_Set) -> s_pos_percent_ETV_Set/1

== system h175_model_cathode_harness_hctrl_basic/Plant_Sensors/EAC_Theo_Power ==
  <mFlow_S1> : Inport
  <aPres_S1> : Inport  Port=2
  <aPres_S2> : Inport  Port=3
  <aTemp_S1> : Inport  Port=4
  Cp : Constant  Value=1004
  Divide : Product  Inputs=*/
  MATLAB Function : MATLAB Function  TreatAsAtomicUnit=on
  Product : Product  Inputs=4
  y-exp : Constant  Value=(1.33-1)/1.33
  Out1 : Outport
  wires:
  Cp/1 -> Product/1
  <aTemp_S1>/1 -> Product/2
  <aPres_S1>/1 -> Divide/2
  Product/1 -> Out1/1
  <aPres_S2>/1 -> Divide/1
  MATLAB Function/1(y) -> Product/4
  y-exp/1 -> MATLAB Function/2(data)
  Divide/1 -> MATLAB Function/1(u)
  <mFlow_S1>/1 -> Product/3

== system h175_model_cathode_harness_hctrl_basic/Plant_Sensors/EAT_Theo_Power ==
  <mFlow_S1> : Inport
  <aPres_S6> : Inport  Port=2
  <aTemp_S6> : Inport  Port=3
  <aPres_S7> : Inport  Port=4
  Cp : Constant  Value=1150
  Divide : Product  Inputs=*/
  Gain : Gain  Gain=-1
  MATLAB Function : MATLAB Function  TreatAsAtomicUnit=on
  Product : Product  Inputs=4
  y-exp : Constant  Value=(1.33-1)/1.33
  Out1 : Outport
  wires:
  y-exp/1 -> MATLAB Function/2(data)
  <aPres_S7>/1 -> Divide/1
  Cp/1 -> Product/4
  Divide/1 -> MATLAB Function/1(u)
  Product/1 -> Gain/1
  <mFlow_S1>/1 -> Product/2
  MATLAB Function/1(y) -> Product/1
  <aTemp_S6>/1 -> Product/3
  <aPres_S6>/1 -> Divide/2
  Gain/1 -> Out1/1

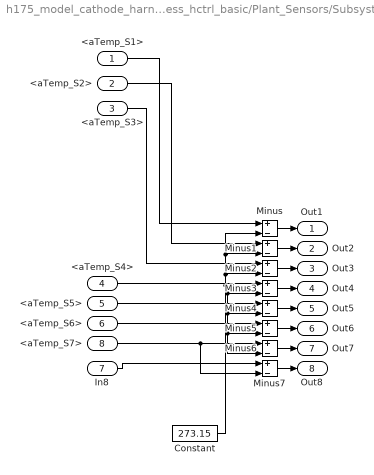
== system h175_model_cathode_harness_hctrl_basic/Plant_Sensors/Subsystem ==
  <aTemp_S1> : Inport
  <aTemp_S2> : Inport  Port=2
  <aTemp_S3> : Inport  Port=3
  <aTemp_S4> : Inport  Port=4
  <aTemp_S5> : Inport  Port=5
  <aTemp_S6> : Inport  Port=6
  In8 : Inport  Port=7
  <aTemp_S7> : Inport  Port=8
  Constant : Constant  Value=273.15
  Minus{,1..7} (8 alike) : Sum  Inputs=+-
  Out1 : Outport
  Out2 : Outport  Port=2
  Out3 : Outport  Port=3
  Out4 : Outport  Port=4
  Out5 : Outport  Port=5
  Out6 : Outport  Port=6
  Out7 : Outport  Port=7
  Out8 : Outport  Port=8
  wires:
  Minus4/1 -> Out5/1
  Constant/1 -> Minus6/2, Minus5/2, Minus4/2, Minus3/2, Minus2/2, Minus1/2, Minus/2
  Minus2/1 -> Out3/1
  <aTemp_S7>/1 -> Minus7/2, Minus6/1
  <aTemp_S4>/1 -> Minus3/1
  <aTemp_S1>/1 -> Minus/1
  Minus5/1 -> Out6/1
  Minus6/1 -> Out7/1
  <aTemp_S3>/1 -> Minus2/1
  Minus/1 -> Out1/1
  <aTemp_S5>/1 -> Minus4/1
  Minus3/1 -> Out4/1
  Minus1/1 -> Out2/1
  <aTemp_S6>/1 -> Minus5/1
  <aTemp_S2>/1 -> Minus1/1
  In8/1 -> Minus7/1
  Minus7/1 -> Out8/1

== system h175_model_cathode_harness_hctrl_basic/Slimmed Down EAC CTRL/FischerWithTurbineControl ==
  s_EAC_mDotSP_gps : Inport
  s_I_A_StN_Get : Inport  Port=2
  s_omega_rpm_EAC_Get : Inport  Port=3
  s_mDot_gps_EACi_Get : Inport  Port=4
  MassflowControlWithTurbine : Subsystem
  PressureControl : Subsystem
  s_omega_rpm_EAC_Set : Outport
  s_pos_percent_ETV_Set : Outport  Port=2
  wires:
  MassflowControlWithTurbine/1(s_EAC_omega_rpm) -> s_omega_rpm_EAC_Set/1
  s_EAC_mDotSP_gps/1 -> MassflowControlWithTurbine/1(s_EAC_mDotSP_gps)
  s_omega_rpm_EAC_Get/1 -> PressureControl/2(s_omega_rpm_EAC_Get)
  PressureControl/1(s_pos_percent_ETV_Set) -> s_pos_percent_ETV_Set/1
  s_mDot_gps_EACi_Get/1 -> MassflowControlWithTurbine/2(s_mDot_gps_EACi_Get)
  s_I_A_StN_Get/1 -> PressureControl/1(s_I_A_StN_Get), MassflowControlWithTurbine/3(s_I_A_StN_Get)

== system h175_model_cathode_harness_hctrl_basic/Slimmed Down EAC CTRL/Subsystem ==
  s_EAC_CurrentState_enum : Inport  PortDimensions=1
  s_EAC_SP_ConstMassflow_mDot_ps : Inport  Port=2  PortDimensions=1
  s_I_A_StN_Get : Inport  Port=3  PortDimensions=1
  Constant : Constant  Value=0  OutDataTypeStr=single
  Multiport Switch1 : MultiPortSwitch  SaturateOnIntegerOverflow=off  InputSameDT=off
  calculation_massflow : Subsystem
  calculation_theoretical_massflow : Subsystem
  interpolate_for_lambdaC : Subsystem
  s_EAC_mDotSP_gps : Outport
  wires:
  Multiport Switch1/1 -> s_EAC_mDotSP_gps/1  "log_EAC_mDotSP_gps"
  interpolate_for_lambdaC/1(s_lambdaC_SP) -> calculation_massflow/2(s_lambdaC_SP)  "log_LambdaC_SP"
  s_I_A_StN_Get/1 -> interpolate_for_lambdaC/1(s_I_A_StN_Get), calculation_theoretical_massflow/1(s_I_A_StN_Get)
  Constant/1 -> Multiport Switch1/4
  calculation_theoretical_massflow/1(s_mDot_0_gps) -> calculation_massflow/1(s_mDot_0_gps)
  s_EAC_SP_ConstMassflow_mDot_ps/1 -> Multiport Switch1/2
  calculation_massflow/1(s_SP_mDot_gps) -> Multiport Switch1/3
  s_EAC_CurrentState_enum/1 -> Multiport Switch1/1

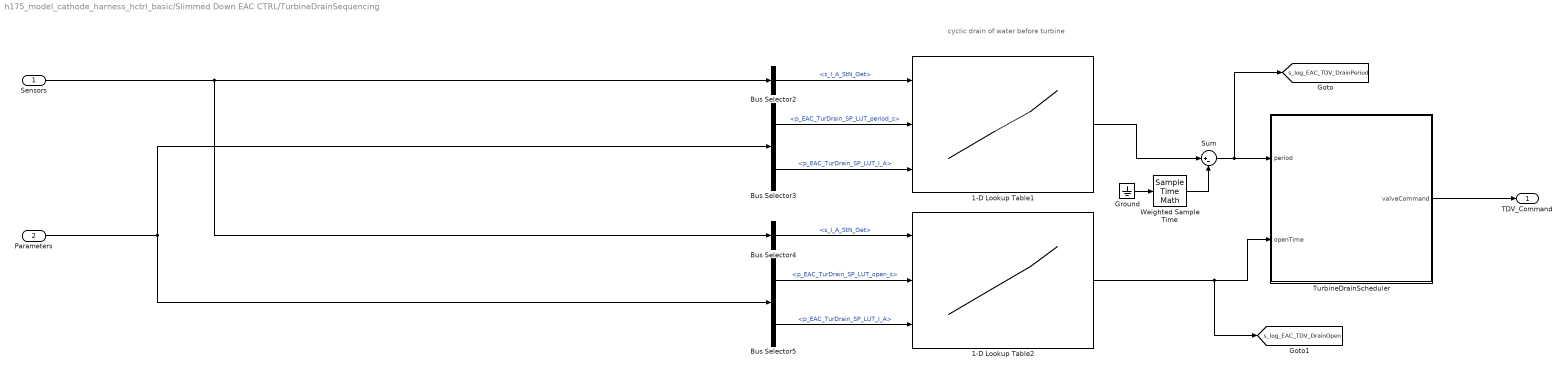
== system h175_model_cathode_harness_hctrl_basic/Slimmed Down EAC CTRL/TurbineDrainSequencing ==
  note: cyclic drain of water before turbine
  Sensors : Inport
  Parameters : Inport  Port=2
  1-D Lookup Table1 : Lookup_n-D  NumberOfTableDimensions=1  BreakpointsForDimension1Source=Input port  BreakpointsForDimension1=[-5:5]  BreakpointsForDimension2Source=Input port  TableSource=Input port  Table=tanh([-5:5])  ExtrapMethod=Clip  InternalRulePriority=Speed  RndMeth=Simplest
      settings: InputPortMap=u0,p221,p5
  1-D Lookup Table2 : Lookup_n-D  NumberOfTableDimensions=1  BreakpointsForDimension1Source=Input port  BreakpointsForDimension1=[-5:5]  BreakpointsForDimension2Source=Input port  TableSource=Input port  Table=tanh([-5:5])  ExtrapMethod=Clip  InternalRulePriority=Speed  RndMeth=Simplest
      settings: InputPortMap=u0,p221,p5
  Bus Selector2 : BusSelector  OutputSignals=b_ElectricalSens.b_Sens_IVT.s_I_A_StN_Get
  Bus Selector3 : BusSelector  OutputSignals=b_CAT_Parameters.b_EAC_Parameters.p_EAC_TurDrain_SP_LUT_period_s,b_CAT_Parameters.b_EAC_Parameters.p_EAC_TurDrain_SP_LUT_I_A
  Bus Selector4 : BusSelector  OutputSignals=b_ElectricalSens.b_Sens_IVT.s_I_A_StN_Get
  Bus Selector5 : BusSelector  OutputSignals=b_CAT_Parameters.b_EAC_Parameters.p_EAC_TurDrain_SP_LUT_open_s,b_CAT_Parameters.b_EAC_Parameters.p_EAC_TurDrain_SP_LUT_I_A
  Ground : Ground
  Sum : Sum  Inputs=|+-
  TurbineDrainScheduler : Stateflow chart  TreatAsAtomicUnit=on
  Weighted Sample Time : SampleTimeMath  TsampMathOp=Ts Only
  TDV_Command : Outport
  tag scope: s_log_EAC_TDV_DrainOpen=global, s_log_EAC_TDV_DrainPeriod=global
  wires:
  Ground/1 -> Weighted Sample Time/1
  TurbineDrainScheduler/1(valveCommand) -> TDV_Command/1
  1-D Lookup Table2/1 -> [s_log_EAC_TDV_DrainOpen], TurbineDrainScheduler/2(openTime)
  Sum/1 -> [s_log_EAC_TDV_DrainPeriod], TurbineDrainScheduler/1(period)
  Weighted Sample Time/1 -> Sum/2
  Sensors/1 -> Bus Selector2/1, Bus Selector4/1
  Bus Selector4/1 -> 1-D Lookup Table2/1  "<s_I_A_StN_Get>"
  Bus Selector3/1 -> 1-D Lookup Table1/2  "<p_EAC_TurDrain_SP_LUT_period_s>"
  Bus Selector3/2 -> 1-D Lookup Table1/3  "<p_EAC_TurDrain_SP_LUT_I_A>"
  1-D Lookup Table1/1 -> Sum/1
  Bus Selector2/1 -> 1-D Lookup Table1/1  "<s_I_A_StN_Get>"
  Parameters/1 -> Bus Selector5/1, Bus Selector3/1
  Bus Selector5/2 -> 1-D Lookup Table2/3  "<p_EAC_TurDrain_SP_LUT_I_A>"
  Bus Selector5/1 -> 1-D Lookup Table2/2  "<p_EAC_TurDrain_SP_LUT_open_s>"

== system h175_model_cathode_harness_hctrl_basic/Slimmed Down EAC CTRL/FischerWithTurbineControl/MassflowControlWithTurbine ==
  s_EAC_mDotSP_gps : Inport
  s_mDot_gps_EACi_Get : Inport  Port=2
  s_I_A_StN_Get : Inport  Port=3
  Add : Sum
  EAC_PID_Feedback_Control : Subsystem
  Subsystem : Subsystem
  s_EAC_omega_rpm : Outport
  wires:
  Add/1 -> s_EAC_omega_rpm/1
  EAC_PID_Feedback_Control/1(s_EAC_PID_omega_rpm) -> Add/2  "s_EAC_PID_omega_rpm"
  Subsystem/1(s_EAC_FF_omega_rpm) -> Add/1, EAC_PID_Feedback_Control/1(s_EAC_FF_omega_rpm)  "s_EAC_FF_omega_rpm"
  s_EAC_mDotSP_gps/1 -> EAC_PID_Feedback_Control/2(s_EAC_mDotSP_gps)
  s_mDot_gps_EACi_Get/1 -> EAC_PID_Feedback_Control/3(s_mDot_gps_EACi_Get)
  s_I_A_StN_Get/1 -> Subsystem/1(s_I_A_StN_Get)

== system h175_model_cathode_harness_hctrl_basic/Slimmed Down EAC CTRL/FischerWithTurbineControl/PressureControl ==
  note: throttle valve position
  s_I_A_StN_Get : Inport
  s_omega_rpm_EAC_Get : Inport  Port=2
  1-D Lookup Table : Lookup_n-D  NumberOfTableDimensions=1  BreakpointsForDimension1=[0 45 100 150 200 250 300 350 400 420 460 500 600]  Table=[100 100 99 98 97 96 95 94 93 92 91 90 89]  ExtrapMethod=Clip  InternalRulePriority=Speed  RndMeth=Simplest
  AlternativeCathodePressureControl : Subsystem  Commented=on
  Multiport Switch : MultiPortSwitch  Commented=on  SaturateOnIntegerOverflow=off  InputSameDT=off
  Sum1 : Sum  Inputs=|++
  SurgeProtection : Subsystem
  s_pos_percent_ETV_Set : Outport
  wires:
  Sum1/1 -> s_pos_percent_ETV_Set/1
  s_omega_rpm_EAC_Get/1 -> SurgeProtection/2(s_EAC_omega_rpm)
  1-D Lookup Table/1 -> Sum1/1
  SurgeProtection/1(SurgeProtectionOpening) -> Sum1/2
  s_I_A_StN_Get/1 -> SurgeProtection/1(s_I_A_StN_Get), 1-D Lookup Table/1

== system h175_model_cathode_harness_hctrl_basic/Slimmed Down EAC CTRL/Subsystem/calculation_massflow ==
  s_mDot_0_gps : Inport
  s_lambdaC_SP : Inport  Port=2
  Product : Product
  s_SP_mDot_gps : Outport
  wires:
  s_mDot_0_gps/1 -> Product/1
  s_lambdaC_SP/1 -> Product/2
  Product/1 -> s_SP_mDot_gps/1

== system h175_model_cathode_harness_hctrl_basic/Slimmed Down EAC CTRL/Subsystem/calculation_theoretical_massflow ==
  s_I_A_StN_Get : Inport
  Cop_NumberOfCellsnstant : Constant  Value=455
  p_Air_O2_Share_Mass_percent : Constant  Value=23.133
  p_FaradaysConstant_AsPerMol : Constant  Value=96485.3399
  p_MolMass_O2_gPerMol : Constant  Value=31.998
  theoretical_massflow : MATLAB Function  TreatAsAtomicUnit=on
  s_mDot_0_gps : Outport
  wires:
  theoretical_massflow/1(s_mDot_0_gps) -> s_mDot_0_gps/1
  Cop_NumberOfCellsnstant/1 -> theoretical_massflow/1(n_cells)
  s_I_A_StN_Get/1 -> theoretical_massflow/5(I_SFC)
  p_MolMass_O2_gPerMol/1 -> theoretical_massflow/2(M_O2)
  p_FaradaysConstant_AsPerMol/1 -> theoretical_massflow/3(F)
  p_Air_O2_Share_Mass_percent/1 -> theoretical_massflow/4(x_m_O2)

== system h175_model_cathode_harness_hctrl_basic/Slimmed Down EAC CTRL/Subsystem/interpolate_for_lambdaC ==
  s_I_A_StN_Get : Inport
  Lambda_C_SP : Lookup_n-D  NumberOfTableDimensions=1  BreakpointsForDimension1="[0      50      100     150     200     250     300     350     400     425     450     475     500]"  Table="[3       3       2.7     2.5     2.3     2.1     1.8     1.7     1.7     1.7     1.7     1.7     1.7]"  ExtrapMethod=Clip  UseLastTableValue=on  InternalRulePriority=Speed  RndMeth=Simplest
  s_lambdaC_SP : Outport
  wires:
  s_I_A_StN_Get/1 -> Lambda_C_SP/1
  Lambda_C_SP/1 -> s_lambdaC_SP/1

== system h175_model_cathode_harness_hctrl_basic/Slimmed Down EAC CTRL/FischerWithTurbineControl/MassflowControlWithTurbine/EAC_PID_Feedback_Control ==
  s_EAC_FF_omega_rpm : Inport
  s_EAC_mDotSP_gps : Inport  Port=2
  s_mDot_gps_EACi_Get : Inport  Port=3
  Discrete PID Controller : slpidlib/PID Controller  Controller=PID  Form=Parallel  TimeDomain=Discrete-time  UseExternalTs=off  SampleTime=-1  IntegratorMethod=Trapezoidal  FilterMethod=Trapezoidal  ControllerParametersSource=internal  P=700  I=400  UseKiTs=off  D=0  N=100  UseFilter=off  TunerSelectOption=Transfer Function Based (PID Tuner App)  InitialConditionSource=internal  InitialConditionForIntegrator=0  InitialConditionForFilter=0  DifferentiatorICPrevScaledInput=0  ExternalReset=none  TrackingMode=off  Kt=1  LimitOutput=on  SatLimitsSource=external  UpperSaturationLimit=inf  LowerSaturationLimit=-inf  LinearizeAsGain=off  AntiWindupMode=clamping  Kb=1  LimitIntegrator=off  UpperIntegratorSaturationLimit=inf  LowerIntegratorSaturationLimit=-inf  POutMin=[]  POutMax=[]  IOutMin=[]  IOutMax=[]  DOutMin=[]  DOutMax=[]  NOutMin=[]  NOutMax=[]  SumOutMin=[]  SumOutMax=[]  SaturationOutMin=[]  SaturationOutMax=[]  PParamMin=[]  PParamMax=[]  IParamMin=[]  IParamMax=[]  DParamMin=[]  DParamMax=[]  NParamMin=[]  NParamMax=[]  KbParamMin=[]  KbParamMax=[]  KtParamMin=[]  KtParamMax=[]  KbOutMin=[]  KbOutMax=[]  KtOutMin=[]  KtOutMax=[]  IntegratorOutMin=[]  IntegratorOutMax=[]  FilterOutMin=[]  FilterOutMax=[]  SumI1OutMin=[]  SumI1OutMax=[]  SumI2OutMin=[]  SumI2OutMax=[]  SumI3OutMin=[]  SumI3OutMax=[]  SumI4OutMin=[]  SumI4OutMax=[]  SumDOutMin=[]  SumDOutMax=[]  DifferentiatorOutMin=[]  DifferentiatorOutMax=[]  FilterDiffOutCoefMin=[]  FilterDiffOutCoefMax=[]  ReciprocalOutMin=[]  ReciprocalOutMax=[]  SumDenOutMin=[]  SumDenOutMax=[]  SumNumOutMin=[]  SumNumOutMax=[]  DivideOutMin=[]  DivideOutMax=[]  UdiffTsProdOutMin=[]  UdiffTsProdOutMax=[]  NTsProdOutMin=[]  NTsProdOutMax=[]  UintegralTsProdOutMin=[]  UintegralTsProdOutMax=[]  UngainTsProdOutMin=[]  UngainTsProdOutMax=[]  ClampingZeroOutDataTypeStr=Inherit: Inherit via back propagation  ClampingZeroOutMin=[]  ClampingZeroOutMax=[]  FilterDenConstantOutDataTypeStr=Inherit: Inherit via back propagation  FilterDenConstantOutMin=[]  FilterDenConstantOutMax=[]  PCopyOutDataTypeStr=Inherit: Inherit via back propagation  PCopyOutMin=[]  PCopyOutMax=[]  NCopyOutDataTypeStr=Inherit: Inherit via back propagation  NCopyOutMin=[]  NCopyOutMax=[]  IntegratorContinuousStateAttributes=''  IntegratorStateMustResolveToSignalObject=off  IntegratorRTWStateStorageClass=Auto  FilterContinuousStateAttributes=''  FilterStateMustResolveToSignalObject=off  FilterRTWStateStorageClass=Auto  ParallelPVariant=InternalParameters  IdealPVariant=Disabled  IVariant=InternalParameters  DVariant=InternalParameters  IntegratorVariant=Discrete  SatVariant=External  AWVariant=DiscClampingParallel  PCopyVariant=Disabled  TRVariant=Disabled  FdbkBlocksVariant=Feedback  IdealPFdbkVariant=Passthrough  SatFdbkVariant=Passthrough  DerivativeFilterVariant=Differentiator  NVariant=Passthrough  NCopyVariant=Disabled_SignalSpec  FilterICVariant=InternalICsDifferentiator  IntegratorICVariant=InternalICs  ExternalResetVariant=Disabled  TRSumVariant=Passthrough  SumFdbkVariant=Enabled  SumVariant=Sum_PID  TsampFilterVariant=InternalTs  TsampNgainVariant=Passthrough  TsampIntegralVariant=Disabled_SignalSpec  ExternalSaturationOutDataTypeStr=Inherit: Same as second input
      settings: LibrarySourceBlock=simulink/Discrete/Discrete PID Controller
  Math Function2 : Math  Operator=reciprocal
  Moving Average (Variable Frequency) : eeGeneralControl/Moving Average (Variable Frequency)  VariantControl=Variant1  LabelModeActiveChoice=Discrete  f0=1/0.5  fmin=1e-3  x0=0  BufferSize=8192  Ts=-1
      settings: LibrarySourceBlock=|
      | ee_sl_lib/General Control/Moving Average
      | (Variable Frequency)
  Sum : Sum  Inputs=|+-
  Sum1 : Sum  Inputs=|+-
  Sum2 : Sum  Inputs=|+-
  p_Fis_EAC_PID_LowerLim_pos_per : Constant  Value=50000
  p_Fis_EAC_PID_UpperLim_pos_per : Constant  Value=120000
  p_Fis_EAC_mDot_Filter_Window_s : Constant  Value=1.7
  s_EAC_PID_omega_rpm : Outport
  wires:
  Discrete PID Controller/1 -> s_EAC_PID_omega_rpm/1  "s_omega_rpm_OUT_EAC"
  Sum/1 -> Discrete PID Controller/1  "e_mDot_gps"
  s_EAC_mDotSP_gps/1 -> Sum/1  "s_EAC_SP_mDotSP_gps"
  s_EAC_FF_omega_rpm/1 -> Sum1/2, Sum2/2
  Sum1/1 -> Discrete PID Controller/2
  Sum2/1 -> Discrete PID Controller/3
  Math Function2/1 -> Moving Average (Variable Frequency)/1
  Moving Average (Variable Frequency)/1 -> Sum/2
  p_Fis_EAC_PID_UpperLim_pos_per/1 -> Sum1/1
  p_Fis_EAC_PID_LowerLim_pos_per/1 -> Sum2/1
  p_Fis_EAC_mDot_Filter_Window_s/1 -> Math Function2/1
  s_mDot_gps_EACi_Get/1 -> Moving Average (Variable Frequency)/2

== system h175_model_cathode_harness_hctrl_basic/Slimmed Down EAC CTRL/FischerWithTurbineControl/MassflowControlWithTurbine/Subsystem ==
  s_I_A_StN_Get : Inport
  LUT_APRV_FF_Current : Lookup_n-D  NumberOfTableDimensions=1  BreakpointsForDimension1="[0    50     100      150     200     250     300     350     400     450]"  Table="[0  50000   50000   63000   76000   86000   95000   105000   109000   113000]"  ExtrapMethod=Clip  UseLastTableValue=on  InternalRulePriority=Speed  RndMeth=Simplest
  s_EAC_FF_omega_rpm : Outport
  wires:
  s_I_A_StN_Get/1 -> LUT_APRV_FF_Current/1
  LUT_APRV_FF_Current/1 -> s_EAC_FF_omega_rpm/1
